simulink model "simulinkTutorial1"  (Simulink 7.7)
settings: Solver=ode45  StartTime=0.0  StopTime=10.0  RelTol=1e-3
libraries: simulink x1
settings Model: Creator=jiannianweng  LastModifiedBy=jiannianweng

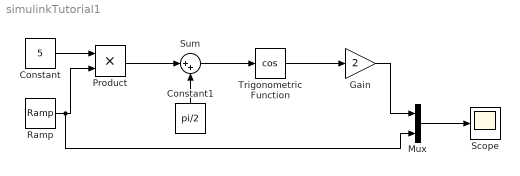
== system simulinkTutorial1 ==
  Constant : Constant  Value=5
  Constant1 : Constant  Value=pi/2
  Gain : Gain  Gain=2
  Mux : Mux  Inputs=2
  Product : Product  RndMeth=Zero
  Ramp : simulink/Sources/Ramp  SystemSampleTime=-1  slope=1  start=0  X0=0
  Scope : Scope
  Sum : Sum  Inputs=|++
  Trigonometric Function : Trigonometry  Operator=cos
  wires:
  Constant/1 -> Product/1
  Ramp/1 -> Product/2, Mux/2
  Constant1/1 -> Sum/2
  Product/1 -> Sum/1
  Sum/1 -> Trigonometric Function/1
  Trigonometric Function/1 -> Gain/1
  Gain/1 -> Mux/1
  Mux/1 -> Scope/1
